simulink model "sim_single_inverted_pendulum"  (R2023a)
settings: Solver=VariableStepAuto  StartTime=0.0  StopTime=5  RelTol=1e-3
settings Model: Creator=ACCENT  LastModifiedBy=ACCENT

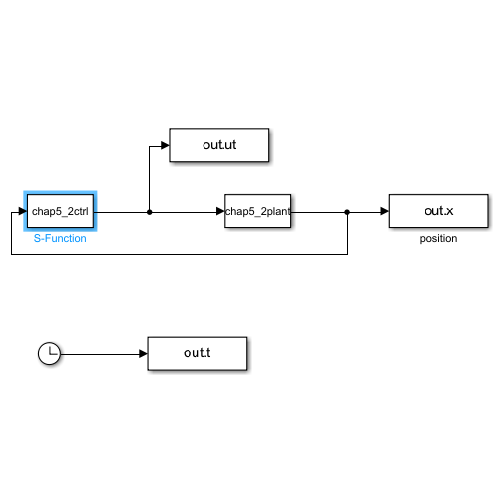
[thumbnail: Simulink's stored preview of the top-level diagram]
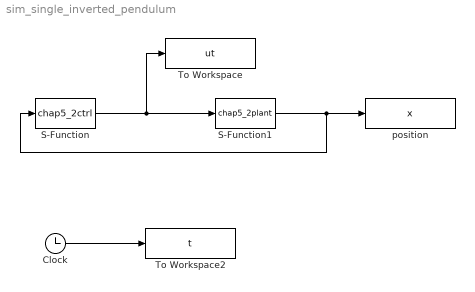
== system sim_single_inverted_pendulum ==
  Clock : Clock
      settings: Decimation=5
  S-Function : S-Function  FunctionName=chap5_2ctrl  SFunctionDeploymentMode=off  EnableBusSupport=off
  S-Function1 : S-Function  FunctionName=chap5_2plant  SFunctionDeploymentMode=off  EnableBusSupport=off
  To Workspace : ToWorkspace  VariableName=ut  SampleTime=-1
  To Workspace2 : ToWorkspace  VariableName=t  SampleTime=-1
  position : ToWorkspace  VariableName=x  SampleTime=-1
  wires:
  Clock/1 -> To Workspace2/1
  S-Function/1 -> To Workspace/1, S-Function1/1
  S-Function1/1 -> S-Function/1, position/1
